simulink model "rx2"  (R2022b)
settings: Solver=FixedStepDiscrete  StartTime=0.0  StopTime=3.3E6  FixedStep=1  RelTol=1e-3  EnableMultiTasking=on
model workspace (MAT data in the model file):
  mwTaskManagerKernelLatency = 0
undefined symbols (not defined in the file or in its folder): Add, jsin, magnitude, rom_pilot_conj_tt, Shift
libraries: hdlsllib x3231, whdlutilities x525, simulink x260, whdlmod x112, whdledac x26, dsphdlmathfun2 x24, commchan3 x1
(part 47 of 59)

== system rx2/process3/decoder/p-p/Subsystem2/Subsystem/Subsystem1/Subsystem ==
  data1 : Inport  OutDataTypeStr=data_type
  wr_addr : Inport  Port=2
  wr_en1 : Inport  Port=3
  rd_addr : Inport  Port=4
  Mux : Mux  Inputs=2
  Selector : Selector  InputPortWidth=8  IndexOptions=Index vector (dialog)  Indices=[1:4]  OutputSizes=1
  Selector1 : Selector  InputPortWidth=8  IndexOptions=Index vector (dialog)  Indices=[5:8]  OutputSizes=1
  Subsystem1 : Subsystem
  Subsystem4 : Subsystem
  rd_dout : Outport  PortDimensions=8  VectorParamsAs1DForOutWhenUnconnected=off
  wires:
  Selector1/1 -> Subsystem1/1(data2)
  Selector/1 -> Subsystem4/1(data2)
  data1/1 -> Selector/1, Selector1/1
  Subsystem1/1(rd_dout1) -> Mux/2
  Subsystem4/1(rd_dout1) -> Mux/1
  Mux/1 -> rd_dout/1
  wr_en1/1 -> Subsystem4/3(wr_en2), Subsystem1/3(wr_en2)
  rd_addr/1 -> Subsystem4/4(rd_addr1), Subsystem1/4(rd_addr1)
  wr_addr/1 -> Subsystem4/2(wr_addr1), Subsystem1/2(wr_addr1)

== system rx2/process3/decoder/p-p/Subsystem2/Subsystem/Subsystem1/Subsystem1 ==
  data1 : Inport  OutDataTypeStr=data_type
  wr_addr : Inport  Port=2
  wr_en1 : Inport  Port=3
  rd_addr : Inport  Port=4
  Mux : Mux  Inputs=2
  Selector : Selector  InputPortWidth=8  IndexOptions=Index vector (dialog)  Indices=[1:4]  OutputSizes=1
  Selector1 : Selector  InputPortWidth=8  IndexOptions=Index vector (dialog)  Indices=[5:8]  OutputSizes=1
  Subsystem1 : Subsystem
  Subsystem4 : Subsystem
  rd_dout : Outport  PortDimensions=8  VectorParamsAs1DForOutWhenUnconnected=off
  wires:
  wr_addr/1 -> Subsystem4/2(wr_addr1), Subsystem1/2(wr_addr1)
  rd_addr/1 -> Subsystem4/4(rd_addr1), Subsystem1/4(rd_addr1)
  wr_en1/1 -> Subsystem4/3(wr_en2), Subsystem1/3(wr_en2)
  Mux/1 -> rd_dout/1
  Subsystem4/1(rd_dout1) -> Mux/1
  Subsystem1/1(rd_dout1) -> Mux/2
  data1/1 -> Selector1/1, Selector/1
  Selector/1 -> Subsystem4/1(data2)
  Selector1/1 -> Subsystem1/1(data2)

== system rx2/process3/decoder/p-p/Subsystem2/Subsystem/Subsystem2/Subsystem ==
  data1 : Inport  OutDataTypeStr=data_type
  wr_addr : Inport  Port=2
  wr_en1 : Inport  Port=3
  rd_addr : Inport  Port=4
  Mux : Mux  Inputs=2
  Selector : Selector  InputPortWidth=8  IndexOptions=Index vector (dialog)  Indices=[1:4]  OutputSizes=1
  Selector1 : Selector  InputPortWidth=8  IndexOptions=Index vector (dialog)  Indices=[5:8]  OutputSizes=1
  Subsystem1 : Subsystem
  Subsystem4 : Subsystem
  rd_dout : Outport  PortDimensions=8  VectorParamsAs1DForOutWhenUnconnected=off
  wires:
  Selector1/1 -> Subsystem1/1(data2)
  Selector/1 -> Subsystem4/1(data2)
  data1/1 -> Selector/1, Selector1/1
  Subsystem1/1(rd_dout1) -> Mux/2
  Subsystem4/1(rd_dout1) -> Mux/1
  Mux/1 -> rd_dout/1
  wr_en1/1 -> Subsystem4/3(wr_en2), Subsystem1/3(wr_en2)
  rd_addr/1 -> Subsystem4/4(rd_addr1), Subsystem1/4(rd_addr1)
  wr_addr/1 -> Subsystem4/2(wr_addr1), Subsystem1/2(wr_addr1)

== system rx2/process3/decoder/p-p/Subsystem2/Subsystem/Subsystem2/Subsystem1 ==
  data1 : Inport  OutDataTypeStr=data_type
  wr_addr : Inport  Port=2
  wr_en1 : Inport  Port=3
  rd_addr : Inport  Port=4
  Mux : Mux  Inputs=2
  Selector : Selector  InputPortWidth=8  IndexOptions=Index vector (dialog)  Indices=[1:4]  OutputSizes=1
  Selector1 : Selector  InputPortWidth=8  IndexOptions=Index vector (dialog)  Indices=[5:8]  OutputSizes=1
  Subsystem1 : Subsystem
  Subsystem4 : Subsystem
  rd_dout : Outport  PortDimensions=8  VectorParamsAs1DForOutWhenUnconnected=off
  wires:
  wr_addr/1 -> Subsystem4/2(wr_addr1), Subsystem1/2(wr_addr1)
  rd_addr/1 -> Subsystem4/4(rd_addr1), Subsystem1/4(rd_addr1)
  wr_en1/1 -> Subsystem4/3(wr_en2), Subsystem1/3(wr_en2)
  Mux/1 -> rd_dout/1
  Subsystem4/1(rd_dout1) -> Mux/1
  Subsystem1/1(rd_dout1) -> Mux/2
  data1/1 -> Selector1/1, Selector/1
  Selector/1 -> Subsystem4/1(data2)
  Selector1/1 -> Subsystem1/1(data2)

== system rx2/process3/decoder/p-p/Subsystem2/Subsystem1/Subsystem1/Subsystem ==
  data1 : Inport  OutDataTypeStr=data_type
  wr_addr : Inport  Port=2
  wr_en1 : Inport  Port=3
  rd_addr : Inport  Port=4
  Mux : Mux  Inputs=2
  Selector : Selector  InputPortWidth=8  IndexOptions=Index vector (dialog)  Indices=[1:4]  OutputSizes=1
  Selector1 : Selector  InputPortWidth=8  IndexOptions=Index vector (dialog)  Indices=[5:8]  OutputSizes=1
  Subsystem1 : Subsystem
  Subsystem4 : Subsystem
  rd_dout : Outport  PortDimensions=8  VectorParamsAs1DForOutWhenUnconnected=off
  wires:
  Selector1/1 -> Subsystem1/1(data2)
  Selector/1 -> Subsystem4/1(data2)
  data1/1 -> Selector/1, Selector1/1
  Subsystem1/1(rd_dout1) -> Mux/2
  Subsystem4/1(rd_dout1) -> Mux/1
  Mux/1 -> rd_dout/1
  wr_en1/1 -> Subsystem4/3(wr_en2), Subsystem1/3(wr_en2)
  rd_addr/1 -> Subsystem4/4(rd_addr1), Subsystem1/4(rd_addr1)
  wr_addr/1 -> Subsystem4/2(wr_addr1), Subsystem1/2(wr_addr1)

== system rx2/process3/decoder/p-p/Subsystem2/Subsystem1/Subsystem1/Subsystem1 ==
  data1 : Inport  OutDataTypeStr=data_type
  wr_addr : Inport  Port=2
  wr_en1 : Inport  Port=3
  rd_addr : Inport  Port=4
  Mux : Mux  Inputs=2
  Selector : Selector  InputPortWidth=8  IndexOptions=Index vector (dialog)  Indices=[1:4]  OutputSizes=1
  Selector1 : Selector  InputPortWidth=8  IndexOptions=Index vector (dialog)  Indices=[5:8]  OutputSizes=1
  Subsystem1 : Subsystem
  Subsystem4 : Subsystem
  rd_dout : Outport  PortDimensions=8  VectorParamsAs1DForOutWhenUnconnected=off
  wires:
  wr_addr/1 -> Subsystem4/2(wr_addr1), Subsystem1/2(wr_addr1)
  rd_addr/1 -> Subsystem4/4(rd_addr1), Subsystem1/4(rd_addr1)
  wr_en1/1 -> Subsystem4/3(wr_en2), Subsystem1/3(wr_en2)
  Mux/1 -> rd_dout/1
  Subsystem4/1(rd_dout1) -> Mux/1
  Subsystem1/1(rd_dout1) -> Mux/2
  data1/1 -> Selector1/1, Selector/1
  Selector/1 -> Subsystem4/1(data2)
  Selector1/1 -> Subsystem1/1(data2)

== system rx2/process3/decoder/p-p/Subsystem2/Subsystem1/Subsystem2/Subsystem ==
  data1 : Inport  OutDataTypeStr=data_type
  wr_addr : Inport  Port=2
  wr_en1 : Inport  Port=3
  rd_addr : Inport  Port=4
  Mux : Mux  Inputs=2
  Selector : Selector  InputPortWidth=8  IndexOptions=Index vector (dialog)  Indices=[1:4]  OutputSizes=1
  Selector1 : Selector  InputPortWidth=8  IndexOptions=Index vector (dialog)  Indices=[5:8]  OutputSizes=1
  Subsystem1 : Subsystem
  Subsystem4 : Subsystem
  rd_dout : Outport  PortDimensions=8  VectorParamsAs1DForOutWhenUnconnected=off
  wires:
  Selector1/1 -> Subsystem1/1(data2)
  Selector/1 -> Subsystem4/1(data2)
  data1/1 -> Selector/1, Selector1/1
  Subsystem1/1(rd_dout1) -> Mux/2
  Subsystem4/1(rd_dout1) -> Mux/1
  Mux/1 -> rd_dout/1
  wr_en1/1 -> Subsystem4/3(wr_en2), Subsystem1/3(wr_en2)
  rd_addr/1 -> Subsystem4/4(rd_addr1), Subsystem1/4(rd_addr1)
  wr_addr/1 -> Subsystem4/2(wr_addr1), Subsystem1/2(wr_addr1)

== system rx2/process3/decoder/p-p/Subsystem2/Subsystem1/Subsystem2/Subsystem1 ==
  data1 : Inport  OutDataTypeStr=data_type
  wr_addr : Inport  Port=2
  wr_en1 : Inport  Port=3
  rd_addr : Inport  Port=4
  Mux : Mux  Inputs=2
  Selector : Selector  InputPortWidth=8  IndexOptions=Index vector (dialog)  Indices=[1:4]  OutputSizes=1
  Selector1 : Selector  InputPortWidth=8  IndexOptions=Index vector (dialog)  Indices=[5:8]  OutputSizes=1
  Subsystem1 : Subsystem
  Subsystem4 : Subsystem
  rd_dout : Outport  PortDimensions=8  VectorParamsAs1DForOutWhenUnconnected=off
  wires:
  wr_addr/1 -> Subsystem4/2(wr_addr1), Subsystem1/2(wr_addr1)
  rd_addr/1 -> Subsystem4/4(rd_addr1), Subsystem1/4(rd_addr1)
  wr_en1/1 -> Subsystem4/3(wr_en2), Subsystem1/3(wr_en2)
  Mux/1 -> rd_dout/1
  Subsystem4/1(rd_dout1) -> Mux/1
  Subsystem1/1(rd_dout1) -> Mux/2
  data1/1 -> Selector1/1, Selector/1
  Selector/1 -> Subsystem4/1(data2)
  Selector1/1 -> Subsystem1/1(data2)

== system rx2/process4/decoder/p-p/Subsystem2/Subsystem/Subsystem1/Subsystem ==
  data1 : Inport  OutDataTypeStr=data_type
  wr_addr : Inport  Port=2
  wr_en1 : Inport  Port=3
  rd_addr : Inport  Port=4
  Mux : Mux  Inputs=2
  Selector : Selector  InputPortWidth=8  IndexOptions=Index vector (dialog)  Indices=[1:4]  OutputSizes=1
  Selector1 : Selector  InputPortWidth=8  IndexOptions=Index vector (dialog)  Indices=[5:8]  OutputSizes=1
  Subsystem1 : Subsystem
  Subsystem4 : Subsystem
  rd_dout : Outport  PortDimensions=8  VectorParamsAs1DForOutWhenUnconnected=off
  wires:
  wr_addr/1 -> Subsystem1/2(wr_addr1), Subsystem4/2(wr_addr1)
  rd_addr/1 -> Subsystem1/4(rd_addr1), Subsystem4/4(rd_addr1)
  wr_en1/1 -> Subsystem1/3(wr_en2), Subsystem4/3(wr_en2)
  Mux/1 -> rd_dout/1
  Subsystem4/1(rd_dout1) -> Mux/1
  Subsystem1/1(rd_dout1) -> Mux/2
  data1/1 -> Selector1/1, Selector/1
  Selector/1 -> Subsystem4/1(data2)
  Selector1/1 -> Subsystem1/1(data2)

== system rx2/process4/decoder/p-p/Subsystem2/Subsystem/Subsystem1/Subsystem1 ==
  data1 : Inport  OutDataTypeStr=data_type
  wr_addr : Inport  Port=2
  wr_en1 : Inport  Port=3
  rd_addr : Inport  Port=4
  Mux : Mux  Inputs=2
  Selector : Selector  InputPortWidth=8  IndexOptions=Index vector (dialog)  Indices=[1:4]  OutputSizes=1
  Selector1 : Selector  InputPortWidth=8  IndexOptions=Index vector (dialog)  Indices=[5:8]  OutputSizes=1
  Subsystem1 : Subsystem
  Subsystem4 : Subsystem
  rd_dout : Outport  PortDimensions=8  VectorParamsAs1DForOutWhenUnconnected=off
  wires:
  Selector1/1 -> Subsystem1/1(data2)
  Selector/1 -> Subsystem4/1(data2)
  data1/1 -> Selector/1, Selector1/1
  Subsystem1/1(rd_dout1) -> Mux/2
  Subsystem4/1(rd_dout1) -> Mux/1
  Mux/1 -> rd_dout/1
  wr_en1/1 -> Subsystem1/3(wr_en2), Subsystem4/3(wr_en2)
  rd_addr/1 -> Subsystem1/4(rd_addr1), Subsystem4/4(rd_addr1)
  wr_addr/1 -> Subsystem1/2(wr_addr1), Subsystem4/2(wr_addr1)

== system rx2/process4/decoder/p-p/Subsystem2/Subsystem/Subsystem2/Subsystem ==
  data1 : Inport  OutDataTypeStr=data_type
  wr_addr : Inport  Port=2
  wr_en1 : Inport  Port=3
  rd_addr : Inport  Port=4
  Mux : Mux  Inputs=2
  Selector : Selector  InputPortWidth=8  IndexOptions=Index vector (dialog)  Indices=[1:4]  OutputSizes=1
  Selector1 : Selector  InputPortWidth=8  IndexOptions=Index vector (dialog)  Indices=[5:8]  OutputSizes=1
  Subsystem1 : Subsystem
  Subsystem4 : Subsystem
  rd_dout : Outport  PortDimensions=8  VectorParamsAs1DForOutWhenUnconnected=off
  wires:
  wr_addr/1 -> Subsystem1/2(wr_addr1), Subsystem4/2(wr_addr1)
  rd_addr/1 -> Subsystem1/4(rd_addr1), Subsystem4/4(rd_addr1)
  wr_en1/1 -> Subsystem1/3(wr_en2), Subsystem4/3(wr_en2)
  Mux/1 -> rd_dout/1
  Subsystem4/1(rd_dout1) -> Mux/1
  Subsystem1/1(rd_dout1) -> Mux/2
  data1/1 -> Selector1/1, Selector/1
  Selector/1 -> Subsystem4/1(data2)
  Selector1/1 -> Subsystem1/1(data2)

== system rx2/process4/decoder/p-p/Subsystem2/Subsystem/Subsystem2/Subsystem1 ==
  data1 : Inport  OutDataTypeStr=data_type
  wr_addr : Inport  Port=2
  wr_en1 : Inport  Port=3
  rd_addr : Inport  Port=4
  Mux : Mux  Inputs=2
  Selector : Selector  InputPortWidth=8  IndexOptions=Index vector (dialog)  Indices=[1:4]  OutputSizes=1
  Selector1 : Selector  InputPortWidth=8  IndexOptions=Index vector (dialog)  Indices=[5:8]  OutputSizes=1
  Subsystem1 : Subsystem
  Subsystem4 : Subsystem
  rd_dout : Outport  PortDimensions=8  VectorParamsAs1DForOutWhenUnconnected=off
  wires:
  Selector1/1 -> Subsystem1/1(data2)
  Selector/1 -> Subsystem4/1(data2)
  data1/1 -> Selector/1, Selector1/1
  Subsystem1/1(rd_dout1) -> Mux/2
  Subsystem4/1(rd_dout1) -> Mux/1
  Mux/1 -> rd_dout/1
  wr_en1/1 -> Subsystem1/3(wr_en2), Subsystem4/3(wr_en2)
  rd_addr/1 -> Subsystem1/4(rd_addr1), Subsystem4/4(rd_addr1)
  wr_addr/1 -> Subsystem1/2(wr_addr1), Subsystem4/2(wr_addr1)

== system rx2/process4/decoder/p-p/Subsystem2/Subsystem1/Subsystem1/Subsystem ==
  data1 : Inport  OutDataTypeStr=data_type
  wr_addr : Inport  Port=2
  wr_en1 : Inport  Port=3
  rd_addr : Inport  Port=4
  Mux : Mux  Inputs=2
  Selector : Selector  InputPortWidth=8  IndexOptions=Index vector (dialog)  Indices=[1:4]  OutputSizes=1
  Selector1 : Selector  InputPortWidth=8  IndexOptions=Index vector (dialog)  Indices=[5:8]  OutputSizes=1
  Subsystem1 : Subsystem
  Subsystem4 : Subsystem
  rd_dout : Outport  PortDimensions=8  VectorParamsAs1DForOutWhenUnconnected=off
  wires:
  wr_addr/1 -> Subsystem1/2(wr_addr1), Subsystem4/2(wr_addr1)
  rd_addr/1 -> Subsystem1/4(rd_addr1), Subsystem4/4(rd_addr1)
  wr_en1/1 -> Subsystem1/3(wr_en2), Subsystem4/3(wr_en2)
  Mux/1 -> rd_dout/1
  Subsystem4/1(rd_dout1) -> Mux/1
  Subsystem1/1(rd_dout1) -> Mux/2
  data1/1 -> Selector1/1, Selector/1
  Selector/1 -> Subsystem4/1(data2)
  Selector1/1 -> Subsystem1/1(data2)

== system rx2/process4/decoder/p-p/Subsystem2/Subsystem1/Subsystem1/Subsystem1 ==
  data1 : Inport  OutDataTypeStr=data_type
  wr_addr : Inport  Port=2
  wr_en1 : Inport  Port=3
  rd_addr : Inport  Port=4
  Mux : Mux  Inputs=2
  Selector : Selector  InputPortWidth=8  IndexOptions=Index vector (dialog)  Indices=[1:4]  OutputSizes=1
  Selector1 : Selector  InputPortWidth=8  IndexOptions=Index vector (dialog)  Indices=[5:8]  OutputSizes=1
  Subsystem1 : Subsystem
  Subsystem4 : Subsystem
  rd_dout : Outport  PortDimensions=8  VectorParamsAs1DForOutWhenUnconnected=off
  wires:
  Selector1/1 -> Subsystem1/1(data2)
  Selector/1 -> Subsystem4/1(data2)
  data1/1 -> Selector/1, Selector1/1
  Subsystem1/1(rd_dout1) -> Mux/2
  Subsystem4/1(rd_dout1) -> Mux/1
  Mux/1 -> rd_dout/1
  wr_en1/1 -> Subsystem1/3(wr_en2), Subsystem4/3(wr_en2)
  rd_addr/1 -> Subsystem1/4(rd_addr1), Subsystem4/4(rd_addr1)
  wr_addr/1 -> Subsystem1/2(wr_addr1), Subsystem4/2(wr_addr1)

== system rx2/process4/decoder/p-p/Subsystem2/Subsystem1/Subsystem2/Subsystem ==
  data1 : Inport  OutDataTypeStr=data_type
  wr_addr : Inport  Port=2
  wr_en1 : Inport  Port=3
  rd_addr : Inport  Port=4
  Mux : Mux  Inputs=2
  Selector : Selector  InputPortWidth=8  IndexOptions=Index vector (dialog)  Indices=[1:4]  OutputSizes=1
  Selector1 : Selector  InputPortWidth=8  IndexOptions=Index vector (dialog)  Indices=[5:8]  OutputSizes=1
  Subsystem1 : Subsystem
  Subsystem4 : Subsystem
  rd_dout : Outport  PortDimensions=8  VectorParamsAs1DForOutWhenUnconnected=off
  wires:
  wr_addr/1 -> Subsystem1/2(wr_addr1), Subsystem4/2(wr_addr1)
  rd_addr/1 -> Subsystem1/4(rd_addr1), Subsystem4/4(rd_addr1)
  wr_en1/1 -> Subsystem1/3(wr_en2), Subsystem4/3(wr_en2)
  Mux/1 -> rd_dout/1
  Subsystem4/1(rd_dout1) -> Mux/1
  Subsystem1/1(rd_dout1) -> Mux/2
  data1/1 -> Selector1/1, Selector/1
  Selector/1 -> Subsystem4/1(data2)
  Selector1/1 -> Subsystem1/1(data2)

== system rx2/process4/decoder/p-p/Subsystem2/Subsystem1/Subsystem2/Subsystem1 ==
  data1 : Inport  OutDataTypeStr=data_type
  wr_addr : Inport  Port=2
  wr_en1 : Inport  Port=3
  rd_addr : Inport  Port=4
  Mux : Mux  Inputs=2
  Selector : Selector  InputPortWidth=8  IndexOptions=Index vector (dialog)  Indices=[1:4]  OutputSizes=1
  Selector1 : Selector  InputPortWidth=8  IndexOptions=Index vector (dialog)  Indices=[5:8]  OutputSizes=1
  Subsystem1 : Subsystem
  Subsystem4 : Subsystem
  rd_dout : Outport  PortDimensions=8  VectorParamsAs1DForOutWhenUnconnected=off
  wires:
  Selector1/1 -> Subsystem1/1(data2)
  Selector/1 -> Subsystem4/1(data2)
  data1/1 -> Selector/1, Selector1/1
  Subsystem1/1(rd_dout1) -> Mux/2
  Subsystem4/1(rd_dout1) -> Mux/1
  Mux/1 -> rd_dout/1
  wr_en1/1 -> Subsystem1/3(wr_en2), Subsystem4/3(wr_en2)
  rd_addr/1 -> Subsystem1/4(rd_addr1), Subsystem4/4(rd_addr1)
  wr_addr/1 -> Subsystem1/2(wr_addr1), Subsystem4/2(wr_addr1)

== system rx2/process5/decoder/p-p/Subsystem2/Subsystem/Subsystem1/Subsystem ==
  data1 : Inport  OutDataTypeStr=data_type
  wr_addr : Inport  Port=2
  wr_en1 : Inport  Port=3
  rd_addr : Inport  Port=4
  Mux : Mux  Inputs=2
  Selector : Selector  InputPortWidth=8  IndexOptions=Index vector (dialog)  Indices=[1:4]  OutputSizes=1
  Selector1 : Selector  InputPortWidth=8  IndexOptions=Index vector (dialog)  Indices=[5:8]  OutputSizes=1
  Subsystem1 : Subsystem
  Subsystem4 : Subsystem
  rd_dout : Outport  PortDimensions=8  VectorParamsAs1DForOutWhenUnconnected=off
  wires:
  Selector1/1 -> Subsystem1/1(data2)
  Selector/1 -> Subsystem4/1(data2)
  data1/1 -> Selector/1, Selector1/1
  Subsystem1/1(rd_dout1) -> Mux/2
  Subsystem4/1(rd_dout1) -> Mux/1
  Mux/1 -> rd_dout/1
  wr_en1/1 -> Subsystem4/3(wr_en2), Subsystem1/3(wr_en2)
  rd_addr/1 -> Subsystem4/4(rd_addr1), Subsystem1/4(rd_addr1)
  wr_addr/1 -> Subsystem4/2(wr_addr1), Subsystem1/2(wr_addr1)

== system rx2/process5/decoder/p-p/Subsystem2/Subsystem/Subsystem1/Subsystem1 ==
  data1 : Inport  OutDataTypeStr=data_type
  wr_addr : Inport  Port=2
  wr_en1 : Inport  Port=3
  rd_addr : Inport  Port=4
  Mux : Mux  Inputs=2
  Selector : Selector  InputPortWidth=8  IndexOptions=Index vector (dialog)  Indices=[1:4]  OutputSizes=1
  Selector1 : Selector  InputPortWidth=8  IndexOptions=Index vector (dialog)  Indices=[5:8]  OutputSizes=1
  Subsystem1 : Subsystem
  Subsystem4 : Subsystem
  rd_dout : Outport  PortDimensions=8  VectorParamsAs1DForOutWhenUnconnected=off
  wires:
  wr_addr/1 -> Subsystem4/2(wr_addr1), Subsystem1/2(wr_addr1)
  rd_addr/1 -> Subsystem4/4(rd_addr1), Subsystem1/4(rd_addr1)
  wr_en1/1 -> Subsystem4/3(wr_en2), Subsystem1/3(wr_en2)
  Mux/1 -> rd_dout/1
  Subsystem4/1(rd_dout1) -> Mux/1
  Subsystem1/1(rd_dout1) -> Mux/2
  data1/1 -> Selector1/1, Selector/1
  Selector/1 -> Subsystem4/1(data2)
  Selector1/1 -> Subsystem1/1(data2)

== system rx2/process5/decoder/p-p/Subsystem2/Subsystem/Subsystem2/Subsystem ==
  data1 : Inport  OutDataTypeStr=data_type
  wr_addr : Inport  Port=2
  wr_en1 : Inport  Port=3
  rd_addr : Inport  Port=4
  Mux : Mux  Inputs=2
  Selector : Selector  InputPortWidth=8  IndexOptions=Index vector (dialog)  Indices=[1:4]  OutputSizes=1
  Selector1 : Selector  InputPortWidth=8  IndexOptions=Index vector (dialog)  Indices=[5:8]  OutputSizes=1
  Subsystem1 : Subsystem
  Subsystem4 : Subsystem
  rd_dout : Outport  PortDimensions=8  VectorParamsAs1DForOutWhenUnconnected=off
  wires:
  Selector1/1 -> Subsystem1/1(data2)
  Selector/1 -> Subsystem4/1(data2)
  data1/1 -> Selector/1, Selector1/1
  Subsystem1/1(rd_dout1) -> Mux/2
  Subsystem4/1(rd_dout1) -> Mux/1
  Mux/1 -> rd_dout/1
  wr_en1/1 -> Subsystem4/3(wr_en2), Subsystem1/3(wr_en2)
  rd_addr/1 -> Subsystem4/4(rd_addr1), Subsystem1/4(rd_addr1)
  wr_addr/1 -> Subsystem4/2(wr_addr1), Subsystem1/2(wr_addr1)

== system rx2/process5/decoder/p-p/Subsystem2/Subsystem/Subsystem2/Subsystem1 ==
  data1 : Inport  OutDataTypeStr=data_type
  wr_addr : Inport  Port=2
  wr_en1 : Inport  Port=3
  rd_addr : Inport  Port=4
  Mux : Mux  Inputs=2
  Selector : Selector  InputPortWidth=8  IndexOptions=Index vector (dialog)  Indices=[1:4]  OutputSizes=1
  Selector1 : Selector  InputPortWidth=8  IndexOptions=Index vector (dialog)  Indices=[5:8]  OutputSizes=1
  Subsystem1 : Subsystem
  Subsystem4 : Subsystem
  rd_dout : Outport  PortDimensions=8  VectorParamsAs1DForOutWhenUnconnected=off
  wires:
  wr_addr/1 -> Subsystem4/2(wr_addr1), Subsystem1/2(wr_addr1)
  rd_addr/1 -> Subsystem4/4(rd_addr1), Subsystem1/4(rd_addr1)
  wr_en1/1 -> Subsystem4/3(wr_en2), Subsystem1/3(wr_en2)
  Mux/1 -> rd_dout/1
  Subsystem4/1(rd_dout1) -> Mux/1
  Subsystem1/1(rd_dout1) -> Mux/2
  data1/1 -> Selector1/1, Selector/1
  Selector/1 -> Subsystem4/1(data2)
  Selector1/1 -> Subsystem1/1(data2)

== system rx2/process5/decoder/p-p/Subsystem2/Subsystem1/Subsystem1/Subsystem ==
  data1 : Inport  OutDataTypeStr=data_type
  wr_addr : Inport  Port=2
  wr_en1 : Inport  Port=3
  rd_addr : Inport  Port=4
  Mux : Mux  Inputs=2
  Selector : Selector  InputPortWidth=8  IndexOptions=Index vector (dialog)  Indices=[1:4]  OutputSizes=1
  Selector1 : Selector  InputPortWidth=8  IndexOptions=Index vector (dialog)  Indices=[5:8]  OutputSizes=1
  Subsystem1 : Subsystem
  Subsystem4 : Subsystem
  rd_dout : Outport  PortDimensions=8  VectorParamsAs1DForOutWhenUnconnected=off
  wires:
  Selector1/1 -> Subsystem1/1(data2)
  Selector/1 -> Subsystem4/1(data2)
  data1/1 -> Selector/1, Selector1/1
  Subsystem1/1(rd_dout1) -> Mux/2
  Subsystem4/1(rd_dout1) -> Mux/1
  Mux/1 -> rd_dout/1
  wr_en1/1 -> Subsystem4/3(wr_en2), Subsystem1/3(wr_en2)
  rd_addr/1 -> Subsystem4/4(rd_addr1), Subsystem1/4(rd_addr1)
  wr_addr/1 -> Subsystem4/2(wr_addr1), Subsystem1/2(wr_addr1)

== system rx2/process5/decoder/p-p/Subsystem2/Subsystem1/Subsystem1/Subsystem1 ==
  data1 : Inport  OutDataTypeStr=data_type
  wr_addr : Inport  Port=2
  wr_en1 : Inport  Port=3
  rd_addr : Inport  Port=4
  Mux : Mux  Inputs=2
  Selector : Selector  InputPortWidth=8  IndexOptions=Index vector (dialog)  Indices=[1:4]  OutputSizes=1
  Selector1 : Selector  InputPortWidth=8  IndexOptions=Index vector (dialog)  Indices=[5:8]  OutputSizes=1
  Subsystem1 : Subsystem
  Subsystem4 : Subsystem
  rd_dout : Outport  PortDimensions=8  VectorParamsAs1DForOutWhenUnconnected=off
  wires:
  wr_addr/1 -> Subsystem4/2(wr_addr1), Subsystem1/2(wr_addr1)
  rd_addr/1 -> Subsystem4/4(rd_addr1), Subsystem1/4(rd_addr1)
  wr_en1/1 -> Subsystem4/3(wr_en2), Subsystem1/3(wr_en2)
  Mux/1 -> rd_dout/1
  Subsystem4/1(rd_dout1) -> Mux/1
  Subsystem1/1(rd_dout1) -> Mux/2
  data1/1 -> Selector1/1, Selector/1
  Selector/1 -> Subsystem4/1(data2)
  Selector1/1 -> Subsystem1/1(data2)

== system rx2/process5/decoder/p-p/Subsystem2/Subsystem1/Subsystem2/Subsystem ==
  data1 : Inport  OutDataTypeStr=data_type
  wr_addr : Inport  Port=2
  wr_en1 : Inport  Port=3
  rd_addr : Inport  Port=4
  Mux : Mux  Inputs=2
  Selector : Selector  InputPortWidth=8  IndexOptions=Index vector (dialog)  Indices=[1:4]  OutputSizes=1
  Selector1 : Selector  InputPortWidth=8  IndexOptions=Index vector (dialog)  Indices=[5:8]  OutputSizes=1
  Subsystem1 : Subsystem
  Subsystem4 : Subsystem
  rd_dout : Outport  PortDimensions=8  VectorParamsAs1DForOutWhenUnconnected=off
  wires:
  Selector1/1 -> Subsystem1/1(data2)
  Selector/1 -> Subsystem4/1(data2)
  data1/1 -> Selector/1, Selector1/1
  Subsystem1/1(rd_dout1) -> Mux/2
  Subsystem4/1(rd_dout1) -> Mux/1
  Mux/1 -> rd_dout/1
  wr_en1/1 -> Subsystem4/3(wr_en2), Subsystem1/3(wr_en2)
  rd_addr/1 -> Subsystem4/4(rd_addr1), Subsystem1/4(rd_addr1)
  wr_addr/1 -> Subsystem4/2(wr_addr1), Subsystem1/2(wr_addr1)

== system rx2/process5/decoder/p-p/Subsystem2/Subsystem1/Subsystem2/Subsystem1 ==
  data1 : Inport  OutDataTypeStr=data_type
  wr_addr : Inport  Port=2
  wr_en1 : Inport  Port=3
  rd_addr : Inport  Port=4
  Mux : Mux  Inputs=2
  Selector : Selector  InputPortWidth=8  IndexOptions=Index vector (dialog)  Indices=[1:4]  OutputSizes=1
  Selector1 : Selector  InputPortWidth=8  IndexOptions=Index vector (dialog)  Indices=[5:8]  OutputSizes=1
  Subsystem1 : Subsystem
  Subsystem4 : Subsystem
  rd_dout : Outport  PortDimensions=8  VectorParamsAs1DForOutWhenUnconnected=off
  wires:
  wr_addr/1 -> Subsystem4/2(wr_addr1), Subsystem1/2(wr_addr1)
  rd_addr/1 -> Subsystem4/4(rd_addr1), Subsystem1/4(rd_addr1)
  wr_en1/1 -> Subsystem4/3(wr_en2), Subsystem1/3(wr_en2)
  Mux/1 -> rd_dout/1
  Subsystem4/1(rd_dout1) -> Mux/1
  Subsystem1/1(rd_dout1) -> Mux/2
  data1/1 -> Selector1/1, Selector/1
  Selector/1 -> Subsystem4/1(data2)
  Selector1/1 -> Subsystem1/1(data2)

== system rx2/process6/decoder/p-p/Subsystem2/Subsystem/Subsystem1/Subsystem ==
  data1 : Inport  OutDataTypeStr=data_type
  wr_addr : Inport  Port=2
  wr_en1 : Inport  Port=3
  rd_addr : Inport  Port=4
  Mux : Mux  Inputs=2
  Selector : Selector  InputPortWidth=8  IndexOptions=Index vector (dialog)  Indices=[1:4]  OutputSizes=1
  Selector1 : Selector  InputPortWidth=8  IndexOptions=Index vector (dialog)  Indices=[5:8]  OutputSizes=1
  Subsystem1 : Subsystem
  Subsystem4 : Subsystem
  rd_dout : Outport  PortDimensions=8  VectorParamsAs1DForOutWhenUnconnected=off
  wires:
  wr_addr/1 -> Subsystem1/2(wr_addr1), Subsystem4/2(wr_addr1)
  rd_addr/1 -> Subsystem1/4(rd_addr1), Subsystem4/4(rd_addr1)
  wr_en1/1 -> Subsystem1/3(wr_en2), Subsystem4/3(wr_en2)
  Mux/1 -> rd_dout/1
  Subsystem4/1(rd_dout1) -> Mux/1
  Subsystem1/1(rd_dout1) -> Mux/2
  data1/1 -> Selector1/1, Selector/1
  Selector/1 -> Subsystem4/1(data2)
  Selector1/1 -> Subsystem1/1(data2)

== system rx2/process6/decoder/p-p/Subsystem2/Subsystem/Subsystem1/Subsystem1 ==
  data1 : Inport  OutDataTypeStr=data_type
  wr_addr : Inport  Port=2
  wr_en1 : Inport  Port=3
  rd_addr : Inport  Port=4
  Mux : Mux  Inputs=2
  Selector : Selector  InputPortWidth=8  IndexOptions=Index vector (dialog)  Indices=[1:4]  OutputSizes=1
  Selector1 : Selector  InputPortWidth=8  IndexOptions=Index vector (dialog)  Indices=[5:8]  OutputSizes=1
  Subsystem1 : Subsystem
  Subsystem4 : Subsystem
  rd_dout : Outport  PortDimensions=8  VectorParamsAs1DForOutWhenUnconnected=off
  wires:
  Selector1/1 -> Subsystem1/1(data2)
  Selector/1 -> Subsystem4/1(data2)
  data1/1 -> Selector/1, Selector1/1
  Subsystem1/1(rd_dout1) -> Mux/2
  Subsystem4/1(rd_dout1) -> Mux/1
  Mux/1 -> rd_dout/1
  wr_en1/1 -> Subsystem1/3(wr_en2), Subsystem4/3(wr_en2)
  rd_addr/1 -> Subsystem1/4(rd_addr1), Subsystem4/4(rd_addr1)
  wr_addr/1 -> Subsystem1/2(wr_addr1), Subsystem4/2(wr_addr1)

== system rx2/process6/decoder/p-p/Subsystem2/Subsystem/Subsystem2/Subsystem ==
  data1 : Inport  OutDataTypeStr=data_type
  wr_addr : Inport  Port=2
  wr_en1 : Inport  Port=3
  rd_addr : Inport  Port=4
  Mux : Mux  Inputs=2
  Selector : Selector  InputPortWidth=8  IndexOptions=Index vector (dialog)  Indices=[1:4]  OutputSizes=1
  Selector1 : Selector  InputPortWidth=8  IndexOptions=Index vector (dialog)  Indices=[5:8]  OutputSizes=1
  Subsystem1 : Subsystem
  Subsystem4 : Subsystem
  rd_dout : Outport  PortDimensions=8  VectorParamsAs1DForOutWhenUnconnected=off
  wires:
  wr_addr/1 -> Subsystem1/2(wr_addr1), Subsystem4/2(wr_addr1)
  rd_addr/1 -> Subsystem1/4(rd_addr1), Subsystem4/4(rd_addr1)
  wr_en1/1 -> Subsystem1/3(wr_en2), Subsystem4/3(wr_en2)
  Mux/1 -> rd_dout/1
  Subsystem4/1(rd_dout1) -> Mux/1
  Subsystem1/1(rd_dout1) -> Mux/2
  data1/1 -> Selector1/1, Selector/1
  Selector/1 -> Subsystem4/1(data2)
  Selector1/1 -> Subsystem1/1(data2)

== system rx2/process6/decoder/p-p/Subsystem2/Subsystem/Subsystem2/Subsystem1 ==
  data1 : Inport  OutDataTypeStr=data_type
  wr_addr : Inport  Port=2
  wr_en1 : Inport  Port=3
  rd_addr : Inport  Port=4
  Mux : Mux  Inputs=2
  Selector : Selector  InputPortWidth=8  IndexOptions=Index vector (dialog)  Indices=[1:4]  OutputSizes=1
  Selector1 : Selector  InputPortWidth=8  IndexOptions=Index vector (dialog)  Indices=[5:8]  OutputSizes=1
  Subsystem1 : Subsystem
  Subsystem4 : Subsystem
  rd_dout : Outport  PortDimensions=8  VectorParamsAs1DForOutWhenUnconnected=off
  wires:
  Selector1/1 -> Subsystem1/1(data2)
  Selector/1 -> Subsystem4/1(data2)
  data1/1 -> Selector/1, Selector1/1
  Subsystem1/1(rd_dout1) -> Mux/2
  Subsystem4/1(rd_dout1) -> Mux/1
  Mux/1 -> rd_dout/1
  wr_en1/1 -> Subsystem1/3(wr_en2), Subsystem4/3(wr_en2)
  rd_addr/1 -> Subsystem1/4(rd_addr1), Subsystem4/4(rd_addr1)
  wr_addr/1 -> Subsystem1/2(wr_addr1), Subsystem4/2(wr_addr1)

== system rx2/process6/decoder/p-p/Subsystem2/Subsystem1/Subsystem1/Subsystem ==
  data1 : Inport  OutDataTypeStr=data_type
  wr_addr : Inport  Port=2
  wr_en1 : Inport  Port=3
  rd_addr : Inport  Port=4
  Mux : Mux  Inputs=2
  Selector : Selector  InputPortWidth=8  IndexOptions=Index vector (dialog)  Indices=[1:4]  OutputSizes=1
  Selector1 : Selector  InputPortWidth=8  IndexOptions=Index vector (dialog)  Indices=[5:8]  OutputSizes=1
  Subsystem1 : Subsystem
  Subsystem4 : Subsystem
  rd_dout : Outport  PortDimensions=8  VectorParamsAs1DForOutWhenUnconnected=off
  wires:
  wr_addr/1 -> Subsystem1/2(wr_addr1), Subsystem4/2(wr_addr1)
  rd_addr/1 -> Subsystem1/4(rd_addr1), Subsystem4/4(rd_addr1)
  wr_en1/1 -> Subsystem1/3(wr_en2), Subsystem4/3(wr_en2)
  Mux/1 -> rd_dout/1
  Subsystem4/1(rd_dout1) -> Mux/1
  Subsystem1/1(rd_dout1) -> Mux/2
  data1/1 -> Selector1/1, Selector/1
  Selector/1 -> Subsystem4/1(data2)
  Selector1/1 -> Subsystem1/1(data2)

== system rx2/process6/decoder/p-p/Subsystem2/Subsystem1/Subsystem1/Subsystem1 ==
  data1 : Inport  OutDataTypeStr=data_type
  wr_addr : Inport  Port=2
  wr_en1 : Inport  Port=3
  rd_addr : Inport  Port=4
  Mux : Mux  Inputs=2
  Selector : Selector  InputPortWidth=8  IndexOptions=Index vector (dialog)  Indices=[1:4]  OutputSizes=1
  Selector1 : Selector  InputPortWidth=8  IndexOptions=Index vector (dialog)  Indices=[5:8]  OutputSizes=1
  Subsystem1 : Subsystem
  Subsystem4 : Subsystem
  rd_dout : Outport  PortDimensions=8  VectorParamsAs1DForOutWhenUnconnected=off
  wires:
  Selector1/1 -> Subsystem1/1(data2)
  Selector/1 -> Subsystem4/1(data2)
  data1/1 -> Selector/1, Selector1/1
  Subsystem1/1(rd_dout1) -> Mux/2
  Subsystem4/1(rd_dout1) -> Mux/1
  Mux/1 -> rd_dout/1
  wr_en1/1 -> Subsystem1/3(wr_en2), Subsystem4/3(wr_en2)
  rd_addr/1 -> Subsystem1/4(rd_addr1), Subsystem4/4(rd_addr1)
  wr_addr/1 -> Subsystem1/2(wr_addr1), Subsystem4/2(wr_addr1)

== system rx2/process6/decoder/p-p/Subsystem2/Subsystem1/Subsystem2/Subsystem ==
  data1 : Inport  OutDataTypeStr=data_type
  wr_addr : Inport  Port=2
  wr_en1 : Inport  Port=3
  rd_addr : Inport  Port=4
  Mux : Mux  Inputs=2
  Selector : Selector  InputPortWidth=8  IndexOptions=Index vector (dialog)  Indices=[1:4]  OutputSizes=1
  Selector1 : Selector  InputPortWidth=8  IndexOptions=Index vector (dialog)  Indices=[5:8]  OutputSizes=1
  Subsystem1 : Subsystem
  Subsystem4 : Subsystem
  rd_dout : Outport  PortDimensions=8  VectorParamsAs1DForOutWhenUnconnected=off
  wires:
  wr_addr/1 -> Subsystem1/2(wr_addr1), Subsystem4/2(wr_addr1)
  rd_addr/1 -> Subsystem1/4(rd_addr1), Subsystem4/4(rd_addr1)
  wr_en1/1 -> Subsystem1/3(wr_en2), Subsystem4/3(wr_en2)
  Mux/1 -> rd_dout/1
  Subsystem4/1(rd_dout1) -> Mux/1
  Subsystem1/1(rd_dout1) -> Mux/2
  data1/1 -> Selector1/1, Selector/1
  Selector/1 -> Subsystem4/1(data2)
  Selector1/1 -> Subsystem1/1(data2)

== system rx2/process6/decoder/p-p/Subsystem2/Subsystem1/Subsystem2/Subsystem1 ==
  data1 : Inport  OutDataTypeStr=data_type
  wr_addr : Inport  Port=2
  wr_en1 : Inport  Port=3
  rd_addr : Inport  Port=4
  Mux : Mux  Inputs=2
  Selector : Selector  InputPortWidth=8  IndexOptions=Index vector (dialog)  Indices=[1:4]  OutputSizes=1
  Selector1 : Selector  InputPortWidth=8  IndexOptions=Index vector (dialog)  Indices=[5:8]  OutputSizes=1
  Subsystem1 : Subsystem
  Subsystem4 : Subsystem
  rd_dout : Outport  PortDimensions=8  VectorParamsAs1DForOutWhenUnconnected=off
  wires:
  Selector1/1 -> Subsystem1/1(data2)
  Selector/1 -> Subsystem4/1(data2)
  data1/1 -> Selector/1, Selector1/1
  Subsystem1/1(rd_dout1) -> Mux/2
  Subsystem4/1(rd_dout1) -> Mux/1
  Mux/1 -> rd_dout/1
  wr_en1/1 -> Subsystem1/3(wr_en2), Subsystem4/3(wr_en2)
  rd_addr/1 -> Subsystem1/4(rd_addr1), Subsystem4/4(rd_addr1)
  wr_addr/1 -> Subsystem1/2(wr_addr1), Subsystem4/2(wr_addr1)

== system rx2/process7/decoder/p-p/Subsystem2/Subsystem/Subsystem1/Subsystem ==
  data1 : Inport  OutDataTypeStr=data_type
  wr_addr : Inport  Port=2
  wr_en1 : Inport  Port=3
  rd_addr : Inport  Port=4
  Mux : Mux  Inputs=2
  Selector : Selector  InputPortWidth=8  IndexOptions=Index vector (dialog)  Indices=[1:4]  OutputSizes=1
  Selector1 : Selector  InputPortWidth=8  IndexOptions=Index vector (dialog)  Indices=[5:8]  OutputSizes=1
  Subsystem1 : Subsystem
  Subsystem4 : Subsystem
  rd_dout : Outport  PortDimensions=8  VectorParamsAs1DForOutWhenUnconnected=off
  wires:
  Selector1/1 -> Subsystem1/1(data2)
  Selector/1 -> Subsystem4/1(data2)
  data1/1 -> Selector/1, Selector1/1
  Subsystem1/1(rd_dout1) -> Mux/2
  Subsystem4/1(rd_dout1) -> Mux/1
  Mux/1 -> rd_dout/1
  wr_en1/1 -> Subsystem4/3(wr_en2), Subsystem1/3(wr_en2)
  rd_addr/1 -> Subsystem4/4(rd_addr1), Subsystem1/4(rd_addr1)
  wr_addr/1 -> Subsystem4/2(wr_addr1), Subsystem1/2(wr_addr1)

== system rx2/process7/decoder/p-p/Subsystem2/Subsystem/Subsystem1/Subsystem1 ==
  data1 : Inport  OutDataTypeStr=data_type
  wr_addr : Inport  Port=2
  wr_en1 : Inport  Port=3
  rd_addr : Inport  Port=4
  Mux : Mux  Inputs=2
  Selector : Selector  InputPortWidth=8  IndexOptions=Index vector (dialog)  Indices=[1:4]  OutputSizes=1
  Selector1 : Selector  InputPortWidth=8  IndexOptions=Index vector (dialog)  Indices=[5:8]  OutputSizes=1
  Subsystem1 : Subsystem
  Subsystem4 : Subsystem
  rd_dout : Outport  PortDimensions=8  VectorParamsAs1DForOutWhenUnconnected=off
  wires:
  wr_addr/1 -> Subsystem4/2(wr_addr1), Subsystem1/2(wr_addr1)
  rd_addr/1 -> Subsystem4/4(rd_addr1), Subsystem1/4(rd_addr1)
  wr_en1/1 -> Subsystem4/3(wr_en2), Subsystem1/3(wr_en2)
  Mux/1 -> rd_dout/1
  Subsystem4/1(rd_dout1) -> Mux/1
  Subsystem1/1(rd_dout1) -> Mux/2
  data1/1 -> Selector1/1, Selector/1
  Selector/1 -> Subsystem4/1(data2)
  Selector1/1 -> Subsystem1/1(data2)

== system rx2/process7/decoder/p-p/Subsystem2/Subsystem/Subsystem2/Subsystem ==
  data1 : Inport  OutDataTypeStr=data_type
  wr_addr : Inport  Port=2
  wr_en1 : Inport  Port=3
  rd_addr : Inport  Port=4
  Mux : Mux  Inputs=2
  Selector : Selector  InputPortWidth=8  IndexOptions=Index vector (dialog)  Indices=[1:4]  OutputSizes=1
  Selector1 : Selector  InputPortWidth=8  IndexOptions=Index vector (dialog)  Indices=[5:8]  OutputSizes=1
  Subsystem1 : Subsystem
  Subsystem4 : Subsystem
  rd_dout : Outport  PortDimensions=8  VectorParamsAs1DForOutWhenUnconnected=off
  wires:
  Selector1/1 -> Subsystem1/1(data2)
  Selector/1 -> Subsystem4/1(data2)
  data1/1 -> Selector/1, Selector1/1
  Subsystem1/1(rd_dout1) -> Mux/2
  Subsystem4/1(rd_dout1) -> Mux/1
  Mux/1 -> rd_dout/1
  wr_en1/1 -> Subsystem4/3(wr_en2), Subsystem1/3(wr_en2)
  rd_addr/1 -> Subsystem4/4(rd_addr1), Subsystem1/4(rd_addr1)
  wr_addr/1 -> Subsystem4/2(wr_addr1), Subsystem1/2(wr_addr1)

== system rx2/process7/decoder/p-p/Subsystem2/Subsystem/Subsystem2/Subsystem1 ==
  data1 : Inport  OutDataTypeStr=data_type
  wr_addr : Inport  Port=2
  wr_en1 : Inport  Port=3
  rd_addr : Inport  Port=4
  Mux : Mux  Inputs=2
  Selector : Selector  InputPortWidth=8  IndexOptions=Index vector (dialog)  Indices=[1:4]  OutputSizes=1
  Selector1 : Selector  InputPortWidth=8  IndexOptions=Index vector (dialog)  Indices=[5:8]  OutputSizes=1
  Subsystem1 : Subsystem
  Subsystem4 : Subsystem
  rd_dout : Outport  PortDimensions=8  VectorParamsAs1DForOutWhenUnconnected=off
  wires:
  wr_addr/1 -> Subsystem4/2(wr_addr1), Subsystem1/2(wr_addr1)
  rd_addr/1 -> Subsystem4/4(rd_addr1), Subsystem1/4(rd_addr1)
  wr_en1/1 -> Subsystem4/3(wr_en2), Subsystem1/3(wr_en2)
  Mux/1 -> rd_dout/1
  Subsystem4/1(rd_dout1) -> Mux/1
  Subsystem1/1(rd_dout1) -> Mux/2
  data1/1 -> Selector1/1, Selector/1
  Selector/1 -> Subsystem4/1(data2)
  Selector1/1 -> Subsystem1/1(data2)

== system rx2/process7/decoder/p-p/Subsystem2/Subsystem1/Subsystem1/Subsystem ==
  data1 : Inport  OutDataTypeStr=data_type
  wr_addr : Inport  Port=2
  wr_en1 : Inport  Port=3
  rd_addr : Inport  Port=4
  Mux : Mux  Inputs=2
  Selector : Selector  InputPortWidth=8  IndexOptions=Index vector (dialog)  Indices=[1:4]  OutputSizes=1
  Selector1 : Selector  InputPortWidth=8  IndexOptions=Index vector (dialog)  Indices=[5:8]  OutputSizes=1
  Subsystem1 : Subsystem
  Subsystem4 : Subsystem
  rd_dout : Outport  PortDimensions=8  VectorParamsAs1DForOutWhenUnconnected=off
  wires:
  Selector1/1 -> Subsystem1/1(data2)
  Selector/1 -> Subsystem4/1(data2)
  data1/1 -> Selector/1, Selector1/1
  Subsystem1/1(rd_dout1) -> Mux/2
  Subsystem4/1(rd_dout1) -> Mux/1
  Mux/1 -> rd_dout/1
  wr_en1/1 -> Subsystem4/3(wr_en2), Subsystem1/3(wr_en2)
  rd_addr/1 -> Subsystem4/4(rd_addr1), Subsystem1/4(rd_addr1)
  wr_addr/1 -> Subsystem4/2(wr_addr1), Subsystem1/2(wr_addr1)

== system rx2/process7/decoder/p-p/Subsystem2/Subsystem1/Subsystem1/Subsystem1 ==
  data1 : Inport  OutDataTypeStr=data_type
  wr_addr : Inport  Port=2
  wr_en1 : Inport  Port=3
  rd_addr : Inport  Port=4
  Mux : Mux  Inputs=2
  Selector : Selector  InputPortWidth=8  IndexOptions=Index vector (dialog)  Indices=[1:4]  OutputSizes=1
  Selector1 : Selector  InputPortWidth=8  IndexOptions=Index vector (dialog)  Indices=[5:8]  OutputSizes=1
  Subsystem1 : Subsystem
  Subsystem4 : Subsystem
  rd_dout : Outport  PortDimensions=8  VectorParamsAs1DForOutWhenUnconnected=off
  wires:
  wr_addr/1 -> Subsystem4/2(wr_addr1), Subsystem1/2(wr_addr1)
  rd_addr/1 -> Subsystem4/4(rd_addr1), Subsystem1/4(rd_addr1)
  wr_en1/1 -> Subsystem4/3(wr_en2), Subsystem1/3(wr_en2)
  Mux/1 -> rd_dout/1
  Subsystem4/1(rd_dout1) -> Mux/1
  Subsystem1/1(rd_dout1) -> Mux/2
  data1/1 -> Selector1/1, Selector/1
  Selector/1 -> Subsystem4/1(data2)
  Selector1/1 -> Subsystem1/1(data2)

== system rx2/process7/decoder/p-p/Subsystem2/Subsystem1/Subsystem2/Subsystem ==
  data1 : Inport  OutDataTypeStr=data_type
  wr_addr : Inport  Port=2
  wr_en1 : Inport  Port=3
  rd_addr : Inport  Port=4
  Mux : Mux  Inputs=2
  Selector : Selector  InputPortWidth=8  IndexOptions=Index vector (dialog)  Indices=[1:4]  OutputSizes=1
  Selector1 : Selector  InputPortWidth=8  IndexOptions=Index vector (dialog)  Indices=[5:8]  OutputSizes=1
  Subsystem1 : Subsystem
  Subsystem4 : Subsystem
  rd_dout : Outport  PortDimensions=8  VectorParamsAs1DForOutWhenUnconnected=off
  wires:
  Selector1/1 -> Subsystem1/1(data2)
  Selector/1 -> Subsystem4/1(data2)
  data1/1 -> Selector/1, Selector1/1
  Subsystem1/1(rd_dout1) -> Mux/2
  Subsystem4/1(rd_dout1) -> Mux/1
  Mux/1 -> rd_dout/1
  wr_en1/1 -> Subsystem4/3(wr_en2), Subsystem1/3(wr_en2)
  rd_addr/1 -> Subsystem4/4(rd_addr1), Subsystem1/4(rd_addr1)
  wr_addr/1 -> Subsystem4/2(wr_addr1), Subsystem1/2(wr_addr1)

== system rx2/process7/decoder/p-p/Subsystem2/Subsystem1/Subsystem2/Subsystem1 ==
  data1 : Inport  OutDataTypeStr=data_type
  wr_addr : Inport  Port=2
  wr_en1 : Inport  Port=3
  rd_addr : Inport  Port=4
  Mux : Mux  Inputs=2
  Selector : Selector  InputPortWidth=8  IndexOptions=Index vector (dialog)  Indices=[1:4]  OutputSizes=1
  Selector1 : Selector  InputPortWidth=8  IndexOptions=Index vector (dialog)  Indices=[5:8]  OutputSizes=1
  Subsystem1 : Subsystem
  Subsystem4 : Subsystem
  rd_dout : Outport  PortDimensions=8  VectorParamsAs1DForOutWhenUnconnected=off
  wires:
  wr_addr/1 -> Subsystem4/2(wr_addr1), Subsystem1/2(wr_addr1)
  rd_addr/1 -> Subsystem4/4(rd_addr1), Subsystem1/4(rd_addr1)
  wr_en1/1 -> Subsystem4/3(wr_en2), Subsystem1/3(wr_en2)
  Mux/1 -> rd_dout/1
  Subsystem4/1(rd_dout1) -> Mux/1
  Subsystem1/1(rd_dout1) -> Mux/2
  data1/1 -> Selector1/1, Selector/1
  Selector/1 -> Subsystem4/1(data2)
  Selector1/1 -> Subsystem1/1(data2)

== system rx2/process8/decoder/p-p/Subsystem2/Subsystem/Subsystem1/Subsystem ==
  data1 : Inport  OutDataTypeStr=data_type
  wr_addr : Inport  Port=2
  wr_en1 : Inport  Port=3
  rd_addr : Inport  Port=4
  Mux : Mux  Inputs=2
  Selector : Selector  InputPortWidth=8  IndexOptions=Index vector (dialog)  Indices=[1:4]  OutputSizes=1
  Selector1 : Selector  InputPortWidth=8  IndexOptions=Index vector (dialog)  Indices=[5:8]  OutputSizes=1
  Subsystem1 : Subsystem
  Subsystem4 : Subsystem
  rd_dout : Outport  PortDimensions=8  VectorParamsAs1DForOutWhenUnconnected=off
  wires:
  wr_addr/1 -> Subsystem1/2(wr_addr1), Subsystem4/2(wr_addr1)
  rd_addr/1 -> Subsystem1/4(rd_addr1), Subsystem4/4(rd_addr1)
  wr_en1/1 -> Subsystem1/3(wr_en2), Subsystem4/3(wr_en2)
  Mux/1 -> rd_dout/1
  Subsystem4/1(rd_dout1) -> Mux/1
  Subsystem1/1(rd_dout1) -> Mux/2
  data1/1 -> Selector1/1, Selector/1
  Selector/1 -> Subsystem4/1(data2)
  Selector1/1 -> Subsystem1/1(data2)

== system rx2/process8/decoder/p-p/Subsystem2/Subsystem/Subsystem1/Subsystem1 ==
  data1 : Inport  OutDataTypeStr=data_type
  wr_addr : Inport  Port=2
  wr_en1 : Inport  Port=3
  rd_addr : Inport  Port=4
  Mux : Mux  Inputs=2
  Selector : Selector  InputPortWidth=8  IndexOptions=Index vector (dialog)  Indices=[1:4]  OutputSizes=1
  Selector1 : Selector  InputPortWidth=8  IndexOptions=Index vector (dialog)  Indices=[5:8]  OutputSizes=1
  Subsystem1 : Subsystem
  Subsystem4 : Subsystem
  rd_dout : Outport  PortDimensions=8  VectorParamsAs1DForOutWhenUnconnected=off
  wires:
  Selector1/1 -> Subsystem1/1(data2)
  Selector/1 -> Subsystem4/1(data2)
  data1/1 -> Selector/1, Selector1/1
  Subsystem1/1(rd_dout1) -> Mux/2
  Subsystem4/1(rd_dout1) -> Mux/1
  Mux/1 -> rd_dout/1
  wr_en1/1 -> Subsystem1/3(wr_en2), Subsystem4/3(wr_en2)
  rd_addr/1 -> Subsystem1/4(rd_addr1), Subsystem4/4(rd_addr1)
  wr_addr/1 -> Subsystem1/2(wr_addr1), Subsystem4/2(wr_addr1)

== system rx2/process8/decoder/p-p/Subsystem2/Subsystem/Subsystem2/Subsystem ==
  data1 : Inport  OutDataTypeStr=data_type
  wr_addr : Inport  Port=2
  wr_en1 : Inport  Port=3
  rd_addr : Inport  Port=4
  Mux : Mux  Inputs=2
  Selector : Selector  InputPortWidth=8  IndexOptions=Index vector (dialog)  Indices=[1:4]  OutputSizes=1
  Selector1 : Selector  InputPortWidth=8  IndexOptions=Index vector (dialog)  Indices=[5:8]  OutputSizes=1
  Subsystem1 : Subsystem
  Subsystem4 : Subsystem
  rd_dout : Outport  PortDimensions=8  VectorParamsAs1DForOutWhenUnconnected=off
  wires:
  wr_addr/1 -> Subsystem1/2(wr_addr1), Subsystem4/2(wr_addr1)
  rd_addr/1 -> Subsystem1/4(rd_addr1), Subsystem4/4(rd_addr1)
  wr_en1/1 -> Subsystem1/3(wr_en2), Subsystem4/3(wr_en2)
  Mux/1 -> rd_dout/1
  Subsystem4/1(rd_dout1) -> Mux/1
  Subsystem1/1(rd_dout1) -> Mux/2
  data1/1 -> Selector1/1, Selector/1
  Selector/1 -> Subsystem4/1(data2)
  Selector1/1 -> Subsystem1/1(data2)

== system rx2/process8/decoder/p-p/Subsystem2/Subsystem/Subsystem2/Subsystem1 ==
  data1 : Inport  OutDataTypeStr=data_type
  wr_addr : Inport  Port=2
  wr_en1 : Inport  Port=3
  rd_addr : Inport  Port=4
  Mux : Mux  Inputs=2
  Selector : Selector  InputPortWidth=8  IndexOptions=Index vector (dialog)  Indices=[1:4]  OutputSizes=1
  Selector1 : Selector  InputPortWidth=8  IndexOptions=Index vector (dialog)  Indices=[5:8]  OutputSizes=1
  Subsystem1 : Subsystem
  Subsystem4 : Subsystem
  rd_dout : Outport  PortDimensions=8  VectorParamsAs1DForOutWhenUnconnected=off
  wires:
  Selector1/1 -> Subsystem1/1(data2)
  Selector/1 -> Subsystem4/1(data2)
  data1/1 -> Selector/1, Selector1/1
  Subsystem1/1(rd_dout1) -> Mux/2
  Subsystem4/1(rd_dout1) -> Mux/1
  Mux/1 -> rd_dout/1
  wr_en1/1 -> Subsystem1/3(wr_en2), Subsystem4/3(wr_en2)
  rd_addr/1 -> Subsystem1/4(rd_addr1), Subsystem4/4(rd_addr1)
  wr_addr/1 -> Subsystem1/2(wr_addr1), Subsystem4/2(wr_addr1)

== system rx2/process8/decoder/p-p/Subsystem2/Subsystem1/Subsystem1/Subsystem ==
  data1 : Inport  OutDataTypeStr=data_type
  wr_addr : Inport  Port=2
  wr_en1 : Inport  Port=3
  rd_addr : Inport  Port=4
  Mux : Mux  Inputs=2
  Selector : Selector  InputPortWidth=8  IndexOptions=Index vector (dialog)  Indices=[1:4]  OutputSizes=1
  Selector1 : Selector  InputPortWidth=8  IndexOptions=Index vector (dialog)  Indices=[5:8]  OutputSizes=1
  Subsystem1 : Subsystem
  Subsystem4 : Subsystem
  rd_dout : Outport  PortDimensions=8  VectorParamsAs1DForOutWhenUnconnected=off
  wires:
  wr_addr/1 -> Subsystem1/2(wr_addr1), Subsystem4/2(wr_addr1)
  rd_addr/1 -> Subsystem1/4(rd_addr1), Subsystem4/4(rd_addr1)
  wr_en1/1 -> Subsystem1/3(wr_en2), Subsystem4/3(wr_en2)
  Mux/1 -> rd_dout/1
  Subsystem4/1(rd_dout1) -> Mux/1
  Subsystem1/1(rd_dout1) -> Mux/2
  data1/1 -> Selector1/1, Selector/1
  Selector/1 -> Subsystem4/1(data2)
  Selector1/1 -> Subsystem1/1(data2)

== system rx2/process8/decoder/p-p/Subsystem2/Subsystem1/Subsystem1/Subsystem1 ==
  data1 : Inport  OutDataTypeStr=data_type
  wr_addr : Inport  Port=2
  wr_en1 : Inport  Port=3
  rd_addr : Inport  Port=4
  Mux : Mux  Inputs=2
  Selector : Selector  InputPortWidth=8  IndexOptions=Index vector (dialog)  Indices=[1:4]  OutputSizes=1
  Selector1 : Selector  InputPortWidth=8  IndexOptions=Index vector (dialog)  Indices=[5:8]  OutputSizes=1
  Subsystem1 : Subsystem
  Subsystem4 : Subsystem
  rd_dout : Outport  PortDimensions=8  VectorParamsAs1DForOutWhenUnconnected=off
  wires:
  Selector1/1 -> Subsystem1/1(data2)
  Selector/1 -> Subsystem4/1(data2)
  data1/1 -> Selector/1, Selector1/1
  Subsystem1/1(rd_dout1) -> Mux/2
  Subsystem4/1(rd_dout1) -> Mux/1
  Mux/1 -> rd_dout/1
  wr_en1/1 -> Subsystem1/3(wr_en2), Subsystem4/3(wr_en2)
  rd_addr/1 -> Subsystem1/4(rd_addr1), Subsystem4/4(rd_addr1)
  wr_addr/1 -> Subsystem1/2(wr_addr1), Subsystem4/2(wr_addr1)

== system rx2/process8/decoder/p-p/Subsystem2/Subsystem1/Subsystem2/Subsystem ==
  data1 : Inport  OutDataTypeStr=data_type
  wr_addr : Inport  Port=2
  wr_en1 : Inport  Port=3
  rd_addr : Inport  Port=4
  Mux : Mux  Inputs=2
  Selector : Selector  InputPortWidth=8  IndexOptions=Index vector (dialog)  Indices=[1:4]  OutputSizes=1
  Selector1 : Selector  InputPortWidth=8  IndexOptions=Index vector (dialog)  Indices=[5:8]  OutputSizes=1
  Subsystem1 : Subsystem
  Subsystem4 : Subsystem
  rd_dout : Outport  PortDimensions=8  VectorParamsAs1DForOutWhenUnconnected=off
  wires:
  wr_addr/1 -> Subsystem1/2(wr_addr1), Subsystem4/2(wr_addr1)
  rd_addr/1 -> Subsystem1/4(rd_addr1), Subsystem4/4(rd_addr1)
  wr_en1/1 -> Subsystem1/3(wr_en2), Subsystem4/3(wr_en2)
  Mux/1 -> rd_dout/1
  Subsystem4/1(rd_dout1) -> Mux/1
  Subsystem1/1(rd_dout1) -> Mux/2
  data1/1 -> Selector1/1, Selector/1
  Selector/1 -> Subsystem4/1(data2)
  Selector1/1 -> Subsystem1/1(data2)

== system rx2/process8/decoder/p-p/Subsystem2/Subsystem1/Subsystem2/Subsystem1 ==
  data1 : Inport  OutDataTypeStr=data_type
  wr_addr : Inport  Port=2
  wr_en1 : Inport  Port=3
  rd_addr : Inport  Port=4
  Mux : Mux  Inputs=2
  Selector : Selector  InputPortWidth=8  IndexOptions=Index vector (dialog)  Indices=[1:4]  OutputSizes=1
  Selector1 : Selector  InputPortWidth=8  IndexOptions=Index vector (dialog)  Indices=[5:8]  OutputSizes=1
  Subsystem1 : Subsystem
  Subsystem4 : Subsystem
  rd_dout : Outport  PortDimensions=8  VectorParamsAs1DForOutWhenUnconnected=off
  wires:
  Selector1/1 -> Subsystem1/1(data2)
  Selector/1 -> Subsystem4/1(data2)
  data1/1 -> Selector/1, Selector1/1
  Subsystem1/1(rd_dout1) -> Mux/2
  Subsystem4/1(rd_dout1) -> Mux/1
  Mux/1 -> rd_dout/1
  wr_en1/1 -> Subsystem1/3(wr_en2), Subsystem4/3(wr_en2)
  rd_addr/1 -> Subsystem1/4(rd_addr1), Subsystem4/4(rd_addr1)
  wr_addr/1 -> Subsystem1/2(wr_addr1), Subsystem4/2(wr_addr1)

== system rx2/process9/decoder/p-p/Subsystem2/Subsystem/Subsystem1/Subsystem ==
  data1 : Inport  OutDataTypeStr=data_type
  wr_addr : Inport  Port=2
  wr_en1 : Inport  Port=3
  rd_addr : Inport  Port=4
  Mux : Mux  Inputs=2
  Selector : Selector  InputPortWidth=8  IndexOptions=Index vector (dialog)  Indices=[1:4]  OutputSizes=1
  Selector1 : Selector  InputPortWidth=8  IndexOptions=Index vector (dialog)  Indices=[5:8]  OutputSizes=1
  Subsystem1 : Subsystem
  Subsystem4 : Subsystem
  rd_dout : Outport  PortDimensions=8  VectorParamsAs1DForOutWhenUnconnected=off
  wires:
  Selector1/1 -> Subsystem1/1(data2)
  Selector/1 -> Subsystem4/1(data2)
  data1/1 -> Selector/1, Selector1/1
  Subsystem1/1(rd_dout1) -> Mux/2
  Subsystem4/1(rd_dout1) -> Mux/1
  Mux/1 -> rd_dout/1
  wr_en1/1 -> Subsystem4/3(wr_en2), Subsystem1/3(wr_en2)
  rd_addr/1 -> Subsystem4/4(rd_addr1), Subsystem1/4(rd_addr1)
  wr_addr/1 -> Subsystem4/2(wr_addr1), Subsystem1/2(wr_addr1)

== system rx2/process9/decoder/p-p/Subsystem2/Subsystem/Subsystem1/Subsystem1 ==
  data1 : Inport  OutDataTypeStr=data_type
  wr_addr : Inport  Port=2
  wr_en1 : Inport  Port=3
  rd_addr : Inport  Port=4
  Mux : Mux  Inputs=2
  Selector : Selector  InputPortWidth=8  IndexOptions=Index vector (dialog)  Indices=[1:4]  OutputSizes=1
  Selector1 : Selector  InputPortWidth=8  IndexOptions=Index vector (dialog)  Indices=[5:8]  OutputSizes=1
  Subsystem1 : Subsystem
  Subsystem4 : Subsystem
  rd_dout : Outport  PortDimensions=8  VectorParamsAs1DForOutWhenUnconnected=off
  wires:
  wr_addr/1 -> Subsystem4/2(wr_addr1), Subsystem1/2(wr_addr1)
  rd_addr/1 -> Subsystem4/4(rd_addr1), Subsystem1/4(rd_addr1)
  wr_en1/1 -> Subsystem4/3(wr_en2), Subsystem1/3(wr_en2)
  Mux/1 -> rd_dout/1
  Subsystem4/1(rd_dout1) -> Mux/1
  Subsystem1/1(rd_dout1) -> Mux/2
  data1/1 -> Selector1/1, Selector/1
  Selector/1 -> Subsystem4/1(data2)
  Selector1/1 -> Subsystem1/1(data2)

== system rx2/process9/decoder/p-p/Subsystem2/Subsystem/Subsystem2/Subsystem ==
  data1 : Inport  OutDataTypeStr=data_type
  wr_addr : Inport  Port=2
  wr_en1 : Inport  Port=3
  rd_addr : Inport  Port=4
  Mux : Mux  Inputs=2
  Selector : Selector  InputPortWidth=8  IndexOptions=Index vector (dialog)  Indices=[1:4]  OutputSizes=1
  Selector1 : Selector  InputPortWidth=8  IndexOptions=Index vector (dialog)  Indices=[5:8]  OutputSizes=1
  Subsystem1 : Subsystem
  Subsystem4 : Subsystem
  rd_dout : Outport  PortDimensions=8  VectorParamsAs1DForOutWhenUnconnected=off
  wires:
  Selector1/1 -> Subsystem1/1(data2)
  Selector/1 -> Subsystem4/1(data2)
  data1/1 -> Selector/1, Selector1/1
  Subsystem1/1(rd_dout1) -> Mux/2
  Subsystem4/1(rd_dout1) -> Mux/1
  Mux/1 -> rd_dout/1
  wr_en1/1 -> Subsystem4/3(wr_en2), Subsystem1/3(wr_en2)
  rd_addr/1 -> Subsystem4/4(rd_addr1), Subsystem1/4(rd_addr1)
  wr_addr/1 -> Subsystem4/2(wr_addr1), Subsystem1/2(wr_addr1)
